simulink model "suspension_system_for_one_wheel"  (R2020b)
settings: Solver=VariableStepAuto  StartTime=0.0  StopTime=100  RelTol=1e-3
PreLoadFcn:
  | t = [0:0.01:10]';
  | Ts = 0.01;
  | stin = [zeros(floor((length(t)/2)+1),1) ; 5*ones(floor(length(t)/2),1)];
  | %t=t';
  | %stin=stin';
model workspace (MAT data in the model file):
  b = 100
  k1 = 2000
  k2 = 2000
  m1 = 200
  m2 = 5
settings Model: Creator=user  LastModifiedBy=user
settings DataIOCC: ExternalInput=[t, stin]  LoadExternalInput=on  SaveFormat=Array  SignalLogging=off  DSMLogging=off  ReturnWorkspaceOutputs=off

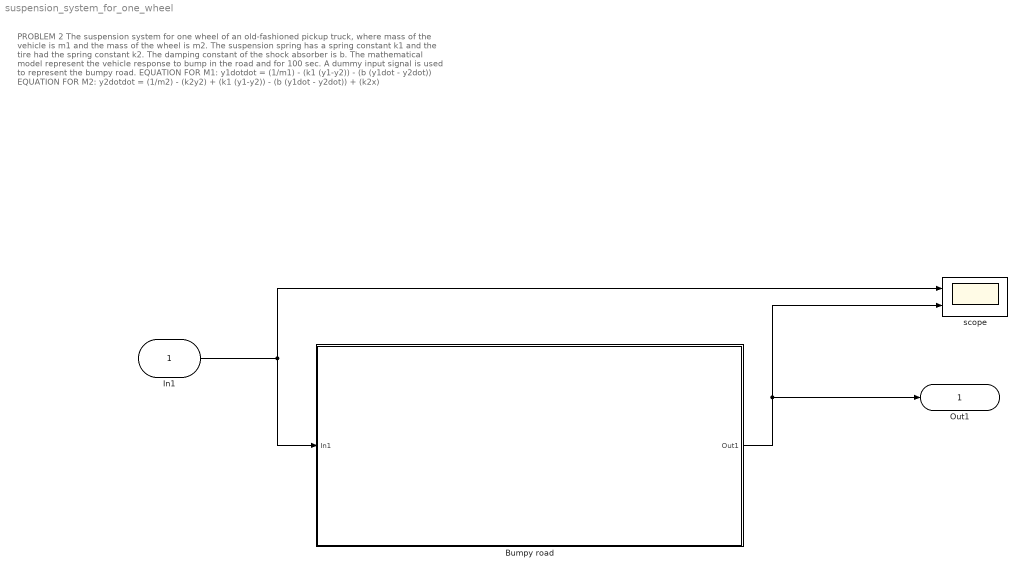
== system suspension_system_for_one_wheel ==
  note: PROBLEM 2
      |
      | The suspension system for one wheel of an old-fashioned pickup truck, where mass of the vehicle is m1 and the mass of the wheel is m2. The suspension spring has a spring constant k1 and the tire had the spring constant k2. The damping constant of the shock absorber is b. The mathematical model represent the vehicle response to bump in the road and for 100 sec. A dummy input signal is used to represent the bumpy road.
      |
      | EQUATION FOR M1:
      | y1dotdot = (1/m1) - (k1 (y1-y2)) - (b (y1dot - y2dot))
      |
      | EQUATION FOR M2:
      | y2dotdot = (1/m2) - (k2y2) + (k1 (y1-y2)) - (b (y1dot - y2dot)) + (k2x)
  In1 : Inport
  " Bumpy road" : Subsystem
      mask Display: image('C:\Users\user\Downloads\Screenshot_20210307-224930.jpg'); % Use "Edit Image" on toolstrip to change.
  scope : Scope  NumInputPorts=2
  Out1 : Outport
  wires:
  " Bumpy road"/1(Out1) -> scope/2, Out1/1
  In1/1 -> scope/1, " Bumpy road"/1(In1)

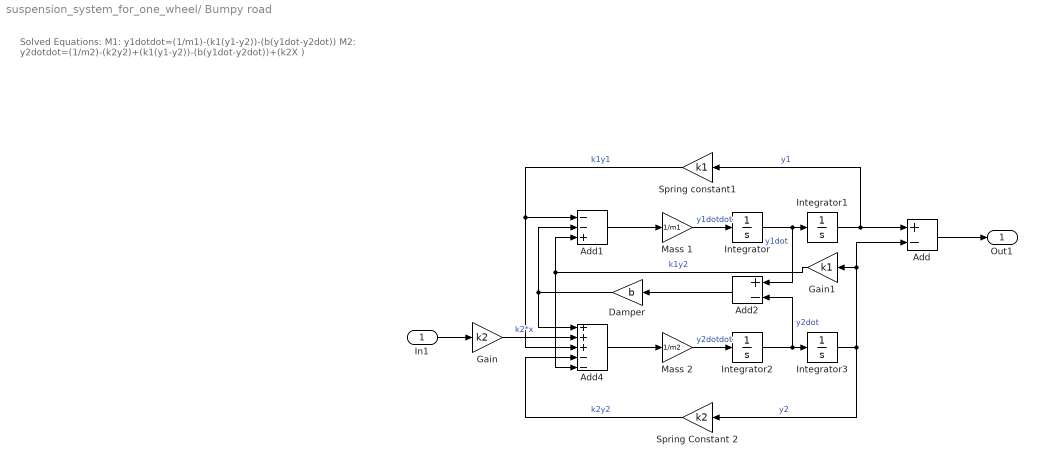
== system suspension_system_for_one_wheel/ Bumpy road ==
  note: Solved Equations:
      |
      | M1:
      | y1dotdot=(1/m1)-(k1(y1-y2))-(b(y1dot-y2dot))
      |
      | M2:
      | y2dotdot=(1/m2)-(k2y2)+(k1(y1-y2))-(b(y1dot-y2dot))+(k2X )
  In1 : Inport
  " Damper" : Gain  Gain=b
  Add : Sum  Inputs=+-
  Add1 : Sum  Inputs=--+
  Add2 : Sum  Inputs=+-
  Add4 : Sum  Inputs=+++--
  Gain : Gain  Gain=k2
  Gain1 : Gain  Gain=k1
  Integrator{,1..3} (4 alike) : Integrator
  Mass 1 : Gain  Gain=1/m1
  Mass 2 : Gain  Gain=1/m2
  Spring Constant 2 : Gain  Gain=k2
  Spring constant1 : Gain  Gain=k1
  Out1 : Outport
  wires:
  Add2/1 -> " Damper"/1
  Spring Constant 2/1 -> Add4/4  "k2y2"
  Integrator3/1 -> Spring Constant 2/1, Gain1/1, Add/2  "y2"
  Add1/1 -> Mass 1/1
  Mass 1/1 -> Integrator/1  "y1dotdot"
  Integrator/1 -> Add2/1, Integrator1/1  "y1dot"
  Integrator2/1 -> Integrator3/1, Add2/2  "y2dot"
  " Damper"/1 -> Add4/1, Add1/2
  Spring constant1/1 -> Add1/1, Add4/3  "k1y1"
  Add/1 -> Out1/1
  Integrator1/1 -> Spring constant1/1, Add/1  "y1"
  Mass 2/1 -> Integrator2/1  "y2dotdot"
  Add4/1 -> Mass 2/1
  In1/1 -> Gain/1
  Gain/1 -> Add4/2  "k2*x"
  Gain1/1 -> Add1/3, Add4/5  "k1y2"
